simulink model "microgrid"  (R2023b)
settings: Solver=VariableStepAuto  StartTime=0.0  StopTime=10.0  RelTol=1e-3
libraries: simulink x10, spsThreePhaseSeriesRLCLoadLib x10, spsThreePhaseBreakerLib x10, spsThreePhaseVIMeasurementLib x6, spsGroundLib x6, eePowerMeasurement x4, spsControlledCurrentSourceLib x3, spsVariableInductorLib x3, spsVariableResistorLib x3, spsThreePhaseSeriesRLCBranchLib x2, spsAsynchronousMachinepuUnitsLib x1, spsThreePhaseTransformerTwoWindingsLib x1
settings Model: Creator=erandum  LastModifiedBy=erandum

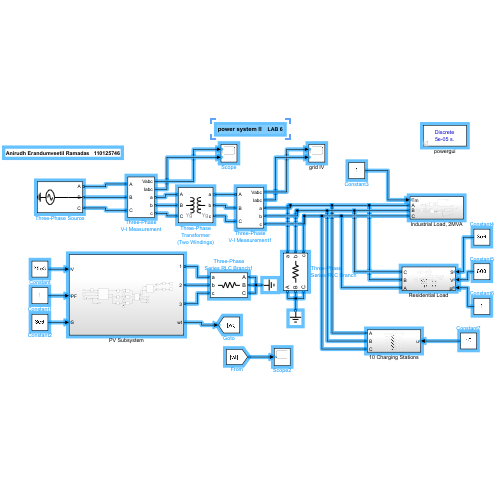
[thumbnail: Simulink's stored preview of the top-level diagram]
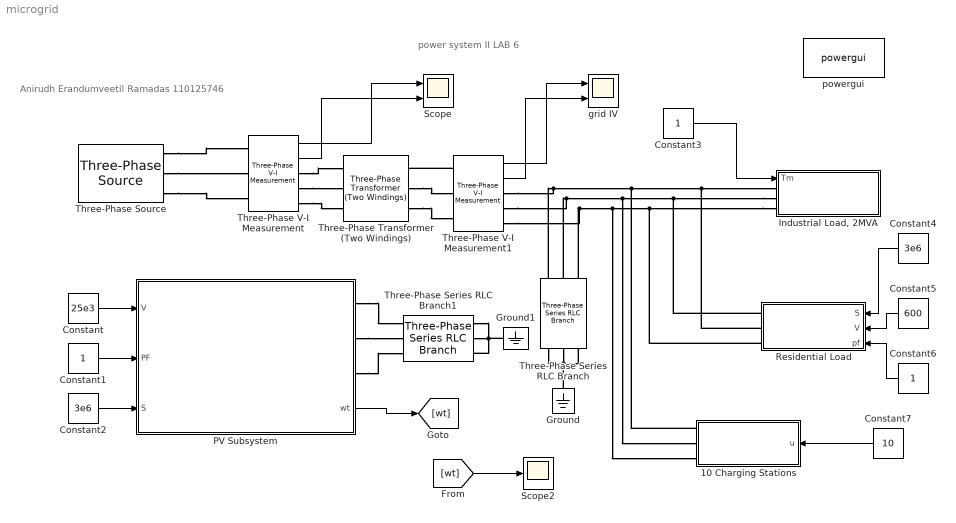
== system microgrid ==
  note: Anirudh Erandumveetil Ramadas 110125746
  note: power system II LAB 6
  10 Charging Stations : Subsystem
      settings: PortSchema="{\"entries\":[{\"content\":{\"sides\":[{\"content\":{\"connectorIds\":[\"LConn1\",\"LConn2\",\"LConn3\"]},\"type\":\"ConnectorPlacement.EquallySpacedRectSide\",\"uuid\":\"f1504b39-5c0e-4613-8c20-d8fb8d5da9a9\"},{\"content\":{\"connectorIds\":[\"In1\"],\"side\":\"RIGHT\"},\"type\":\"ConnectorPlacement.EquallySpacedRectSide\",\"uuid\":\"95b16e74-2cd8-4ce2-9ea5-c38ee840ee39\"},{\"content\":{\"side\":\"TOP\"},\"type\":\"ConnectorPlacement.EquallySpacedRectSide\",\"uuid\":\"c0d1c360-d2d5-4b2e-94da-07f0205a169d\"}]},\"type\":\"ConnectorPlacement.EquallySpacedConnector\",\"uuid\":\"27e98b22-6a64-4901-bf78-f4c065c24ca2\"}],\"packageUris\":[\"http://schema.mathworks.com/mf0/Connector/R2020b\"],\"version\":\"1.0\"}"
  Constant : Constant  Value=25e3
  Constant1 : Constant
  Constant2 : Constant  Value=3e6
  Constant3 : Constant
  Constant4 : Constant  Value=3e6
  Constant5 : Constant  Value=600
  Constant6 : Constant
  Constant7 : Constant  Value=10
  Ground : spsGroundLib/Ground  LConnTagsString=a
  Ground1 : spsGroundLib/Ground  LConnTagsString=a
  "Industrial Load, 2MVA" : Subsystem
  PV Subsystem : Subsystem
      settings: PortSchema="{\"entries\":[{\"content\":{\"sides\":[{\"content\":{\"connectorIds\":[\"In1\",\"In2\",\"In3\"]},\"type\":\"ConnectorPlacement.EquallySpacedRectSide\",\"uuid\":\"95cd3cc3-0877-4a04-ab5d-22b0c69ea079\"},{\"content\":{\"connectorIds\":[\"RConn1\",\"RConn2\",\"RConn3\",\"Out1\"],\"side\":\"RIGHT\"},\"type\":\"ConnectorPlacement.EquallySpacedRectSide\",\"uuid\":\"49167ea2-c585-4edc-b110-423b60a28fbc\"},{\"content\":{\"side\":\"TOP\"},\"type\":\"ConnectorPlacement.EquallySpacedRectSide\",\"uuid\":\"ee5ad331-2692-438a-a456-e1cd48d871f3\"}]},\"type\":\"ConnectorPlacement.EquallySpacedConnector\",\"uuid\":\"ab25702f-315c-43d0-b963-a7196bf7c14e\"}],\"packageUris\":[\"http://schema.mathworks.com/mf0/Connector/R2020b\"],\"version\":\"1.0\"}"
  Residential Load : Subsystem
      settings: PortSchema="{\"entries\":[{\"content\":{\"sides\":[{\"content\":{\"connectorIds\":[\"LConn1\",\"LConn2\",\"LConn3\"]},\"type\":\"ConnectorPlacement.EquallySpacedRectSide\",\"uuid\":\"1b5f4c68-a4bb-47ef-ac05-1fe32ae0a57a\"},{\"content\":{\"connectorIds\":[\"In1\",\"In2\",\"In3\"],\"side\":\"RIGHT\"},\"type\":\"ConnectorPlacement.EquallySpacedRectSide\",\"uuid\":\"b4b4f3e1-57b7-439b-8804-ae777d4c8250\"},{\"content\":{\"side\":\"TOP\"},\"type\":\"ConnectorPlacement.EquallySpacedRectSide\",\"uuid\":\"ef7d5d17-74d1-4089-bbe8-687aade085af\"}]},\"type\":\"ConnectorPlacement.EquallySpacedConnector\",\"uuid\":\"123b8064-54c2-4dec-b119-44036af93a53\"}],\"packageUris\":[\"http://schema.mathworks.com/mf0/Connector/R2020b\"],\"version\":\"1.0\"}"
  Scope : Scope  NumInputPorts=2
  Scope2 : Scope
  Three-Phase Series RLC Branch : spsThreePhaseSeriesRLCBranchLib/Three-Phase Series RLC Branch  LConnTagsString=A|B|C  RConnTagsString=A|B|C  BranchType=R  Resistance=1e6  Inductance=1e-3  Capacitance=1e-6  Measurements=None
  Three-Phase Series RLC Branch1 : spsThreePhaseSeriesRLCBranchLib/Three-Phase Series RLC Branch  LConnTagsString=A|B|C  RConnTagsString=A|B|C  BranchType=R  Resistance=1e6  Inductance=1e-3  Capacitance=1e-6  Measurements=None
  Three-Phase Transformer (Two Windings) : spsThreePhaseTransformerTwoWindingsLib/Three-Phase Transformer (Two Windings)  Winding1Connection=Yg  Winding2Connection=Yg  CoreType=Three single-phase transformers  SetSaturation=off  Hysteresis=off  DataFile='hysteresis'  SetInitialFlux=off  Measurements=None  UNITS=pu  NominalPower=[ 20e6 , 60 ]  Winding1=[ 25e3 , 0.002 , 0.08 ]  Winding2=[ 630 , 0.002 , 0.08 ]  Rm=500  Lm=500  L0=0.5  Saturation=[ 0,0 ; 0.0024,1.2 ; 1.0,1.52 ]  InitialFluxes=[ 0.8 , -0.8 , 0.7 ]  BreakLoop=off  DiscreteSolver=Trapezoidal iterative  DataType=off  TransfoNumber=1
  Three-Phase V-I Measurement : spsThreePhaseVIMeasurementLib/Three-Phase V-I Measurement  VoltageMeasurement=phase-to-ground  SetLabelV=off  LabelV=Vabc  Vpu=off  VpuLL=off  CurrentMeasurement=yes  SetLabelI=off  LabelI=Iabc  Ipu=off  Pbase=100e6  Vbase=500e3  OutputType=Complex  PhasorSimulation=off  PSBequivalent=0
  Three-Phase V-I Measurement1 : spsThreePhaseVIMeasurementLib/Three-Phase V-I Measurement  VoltageMeasurement=phase-to-ground  SetLabelV=off  LabelV=Vabc  Vpu=off  VpuLL=off  CurrentMeasurement=yes  SetLabelI=off  LabelI=Iabc  Ipu=off  Pbase=100e6  Vbase=500e3  OutputType=Complex  PhasorSimulation=off  PSBequivalent=0
  Three-Phase Source : spsThreePhaseSourceLib/Three-Phase Source  InternalConnection=Yg  VoltagePhases=off  Voltage=25e3  PhaseAngle=0  Voltage_phases=[25e3 25e3 25e3]/sqrt(3)  PhaseAngles_phases=[0 -120 +120]  Frequency=60  NonIdealSource=on  SpecifyImpedance=off  Resistance=0  Inductance=0  ShortCircuitLevel=100e6  BaseVoltage=25e3  XRratio=7  BusType=swing  Pref=10e3  Qref=0  Prefabc=[10e3, 10e3, 10e3]  Qrefabc=[0, 0, 0]  Qmin=-inf  Qmax=inf
  grid IV : Scope  NumInputPorts=2
  powergui : sps_lib/powergui  Priority=1  SimulationMode=Discrete  SampleTime=5e-05  frequency=60  Iterations=50  frequencyindice=0  Pbase=100e6  ErrMax=1e-4  UnitsV=kV  UnitsW=MW  buscounter=0  FunctionMessages=off  echomessages=off  EnableUseOfTLC=off  CurrentSourceSwitches=off  DisableSnubberDevices=off  DisableRonSwitches=off  DisableVfSwitches=off  DisplayEquations=off  AutomaticDiscreteSolvers=off  SolverType=Tustin/Backward Euler (TBE)  Interpol=off  ExternalGateDelay=off  methode=off  Ts=100  x0status=blocks  SPID=on  SwTol=0  HookPort=off  NonlinearTolerance=1e-4  nMaxIteration=100  ContinueOnMaxIteration=off  RestoreLinks=warning  ResistiveCurrentMeasurement=off  Frange=[0:2:500]  Ylog=off  Xlog=on  ShowGrid=off  save=off  variable=ZData  structure=0  ZoomFFT=off  StartTime=0.0  cycles=1  DisplayStyle=1  fundamental=60  FreqAxis=off  MaxFrequency=1000  frequencyindicesteady=1  RmsSteady=1  display=off
  wires:
  PV Subsystem/1(wt) -> [wt]
  Constant5/1 -> Residential Load/2(V)
  Constant3/1 -> "Industrial Load, 2MVA"/1(Tm)
  [wt] -> Scope2/1
  Constant4/1 -> Residential Load/1(S)
  Three-Phase V-I Measurement1/2 -> grid IV/2
  Three-Phase V-I Measurement1/1 -> grid IV/1
  Three-Phase V-I Measurement/2 -> Scope/2
  Constant7/1 -> 10 Charging Stations/1(u)
  Constant/1 -> PV Subsystem/1(V)
  Constant6/1 -> Residential Load/3(pf)
  Three-Phase V-I Measurement/1 -> Scope/1
  Constant2/1 -> PV Subsystem/3(S)
  Constant1/1 -> PV Subsystem/2(PF)
  connections:
  "Industrial Load, 2MVA"/LConn3 -- Three-Phase V-I Measurement1/RConn3 -- Three-Phase Series RLC Branch/RConn3 -- 10 Charging Stations/LConn3 -- Residential Load/LConn3
  "Industrial Load, 2MVA"/LConn2 -- Residential Load/LConn1 -- Three-Phase V-I Measurement1/RConn2 -- Three-Phase Series RLC Branch/RConn2 -- 10 Charging Stations/LConn2
  Three-Phase Series RLC Branch/RConn1 -- Three-Phase V-I Measurement1/RConn1 -- 10 Charging Stations/LConn1 -- Residential Load/LConn2 -- "Industrial Load, 2MVA"/LConn1
  Three-Phase Series RLC Branch/LConn2 -- Three-Phase Series RLC Branch/LConn1 -- Three-Phase Series RLC Branch/LConn3 -- Ground/LConn1
  Three-Phase Series RLC Branch1/LConn3 -- Three-Phase Series RLC Branch1/LConn1 -- Ground1/LConn1 -- Three-Phase Series RLC Branch1/LConn2
  PV Subsystem/RConn3 -- Three-Phase Series RLC Branch1/RConn3
  Three-Phase V-I Measurement/RConn1 -- Three-Phase Transformer (Two Windings)/LConn1
  PV Subsystem/RConn2 -- Three-Phase Series RLC Branch1/RConn2
  Three-Phase V-I Measurement/RConn2 -- Three-Phase Transformer (Two Windings)/LConn2
  Three-Phase Source/RConn3 -- Three-Phase V-I Measurement/LConn3
  Three-Phase V-I Measurement1/LConn1 -- Three-Phase Transformer (Two Windings)/RConn1
  Three-Phase Transformer (Two Windings)/RConn2 -- Three-Phase V-I Measurement1/LConn2
  Three-Phase Transformer (Two Windings)/RConn3 -- Three-Phase V-I Measurement1/LConn3
  Three-Phase Source/RConn1 -- Three-Phase V-I Measurement/LConn1
  PV Subsystem/RConn1 -- Three-Phase Series RLC Branch1/RConn1
  Three-Phase Source/RConn2 -- Three-Phase V-I Measurement/LConn2
  Three-Phase V-I Measurement/RConn3 -- Three-Phase Transformer (Two Windings)/LConn3

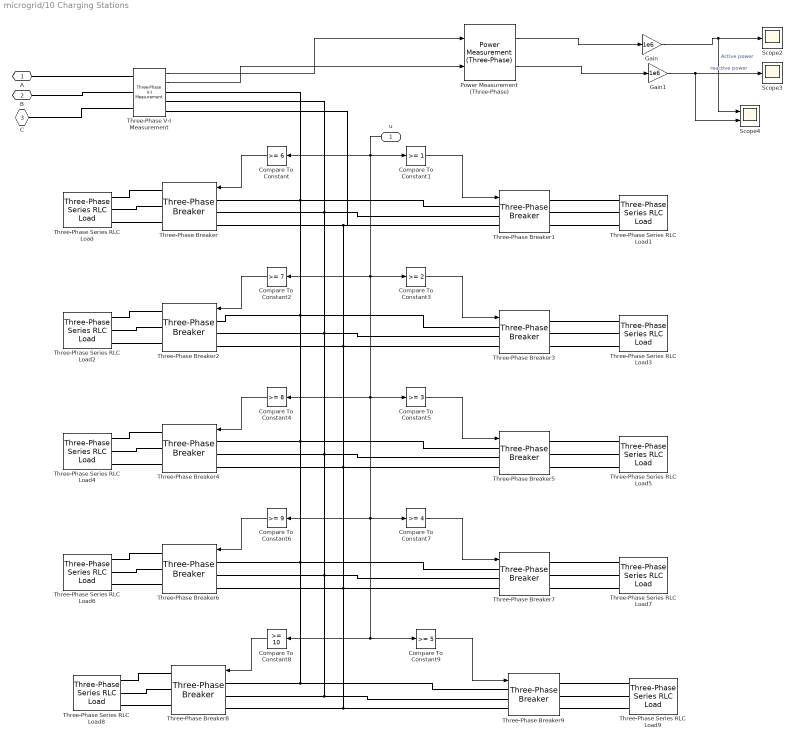
== system microgrid/10 Charging Stations ==
  u : Inport
  Compare To Constant : simulink/Logic and Bit Operations/Compare To Constant  relop=>=  const=6  OutDataTypeStr=boolean
  Compare To Constant1 : simulink/Logic and Bit Operations/Compare To Constant  relop=>=  const=1  OutDataTypeStr=boolean
  Compare To Constant2 : simulink/Logic and Bit Operations/Compare To Constant  relop=>=  const=7  OutDataTypeStr=boolean
  Compare To Constant3 : simulink/Logic and Bit Operations/Compare To Constant  relop=>=  const=2  OutDataTypeStr=boolean
  Compare To Constant4 : simulink/Logic and Bit Operations/Compare To Constant  relop=>=  const=8  OutDataTypeStr=boolean
  Compare To Constant5 : simulink/Logic and Bit Operations/Compare To Constant  relop=>=  const=3  OutDataTypeStr=boolean
  Compare To Constant6 : simulink/Logic and Bit Operations/Compare To Constant  relop=>=  const=9  OutDataTypeStr=boolean
  Compare To Constant7 : simulink/Logic and Bit Operations/Compare To Constant  relop=>=  const=4  OutDataTypeStr=boolean
  Compare To Constant8 : simulink/Logic and Bit Operations/Compare To Constant  relop=>=  const=10  OutDataTypeStr=boolean
  Compare To Constant9 : simulink/Logic and Bit Operations/Compare To Constant  relop=>=  const=5  OutDataTypeStr=boolean
  Gain : Gain  Gain=1e6
  Gain1 : Gain  Gain=1e6
  Power Measurement (Three-Phase) : eePowerMeasurement/Power Measurement (Three-Phase)  LabelModeActiveChoice=Continuous  F=60  K=[0 1 2 3]  Seq=Positive  Ts=0
  Scope2 : Scope
  Scope3 : Scope
  Scope4 : Scope  NumInputPorts=2
  Three-Phase Series RLC Load{,1..9} (10 alike) : spsThreePhaseSeriesRLCLoadLib/Three-Phase Series RLC Load  LConnTagsString=A|B|C  Configuration=Y (grounded)  NominalVoltage=600  Vabc=[1e3 1e3 1e3]  Vabcp=[1e3 1e3 1e3]  NominalFrequency=60  UnbalancedPower=off  ActivePower=400e3  InductivePower=0  CapacitivePower=0  Pabc=[10e3 9e3 11e3]  QLabc=[100 90 110]  QCabc=[100 90 110]  Pabcp=[10e3 9e3 11e3]  QLabcp=[100 90 110]  QCabcp=[100 90 110]  Measurements=None  LoadType=constant Z
  Three-Phase V-I Measurement : spsThreePhaseVIMeasurementLib/Three-Phase V-I Measurement  VoltageMeasurement=phase-to-ground  SetLabelV=off  LabelV=Vabc  Vpu=off  VpuLL=off  CurrentMeasurement=yes  SetLabelI=off  LabelI=Iabc  Ipu=off  Pbase=100e6  Vbase=500e3  OutputType=Complex  PhasorSimulation=off  PSBequivalent=0
  Three-Phase Breaker{,1..9} (10 alike) : spsThreePhaseBreakerLib/Three-Phase Breaker  InitialState=open  SwitchA=on  SwitchB=on  SwitchC=on  SwitchTimes="[1/60  5/60]"  External=on  BreakerResistance=0.01  SnubberResistance=1e6  SnubberCapacitance=inf  Measurements=None
  A : PMIOPort  Side=Left
  B : PMIOPort  Port=2  Side=Left
  C : PMIOPort  Port=3  Side=Left
  wires:
  Compare To Constant/1 -> Three-Phase Breaker/1
  Compare To Constant1/1 -> Three-Phase Breaker1/1
  Compare To Constant3/1 -> Three-Phase Breaker3/1
  Compare To Constant2/1 -> Three-Phase Breaker2/1
  Compare To Constant5/1 -> Three-Phase Breaker5/1
  Compare To Constant4/1 -> Three-Phase Breaker4/1
  Compare To Constant7/1 -> Three-Phase Breaker7/1
  Compare To Constant6/1 -> Three-Phase Breaker6/1
  Compare To Constant9/1 -> Three-Phase Breaker9/1
  Compare To Constant8/1 -> Three-Phase Breaker8/1
  u/1 -> Compare To Constant4/1, Compare To Constant5/1, Compare To Constant6/1, Compare To Constant7/1, Compare To Constant8/1, Compare To Constant9/1, Compare To Constant2/1, Compare To Constant3/1, Compare To Constant/1, Compare To Constant1/1
  Three-Phase V-I Measurement/1 -> Power Measurement (Three-Phase)/1
  Three-Phase V-I Measurement/2 -> Power Measurement (Three-Phase)/2
  Gain/1 -> Scope4/1, Scope2/1  "Active power"
  Gain1/1 -> Scope4/2, Scope3/1  "reactive power"
  Power Measurement (Three-Phase)/1 -> Gain/1
  Power Measurement (Three-Phase)/2 -> Gain1/1
  connections:
  A/RConn1 -- Three-Phase V-I Measurement/LConn1
  B/RConn1 -- Three-Phase V-I Measurement/LConn2
  C/RConn1 -- Three-Phase V-I Measurement/LConn3
  Three-Phase Series RLC Load/LConn1 -- Three-Phase Breaker/RConn1
  Three-Phase Series RLC Load/LConn2 -- Three-Phase Breaker/RConn2
  Three-Phase Series RLC Load/LConn3 -- Three-Phase Breaker/RConn3
  Three-Phase Breaker9/LConn1 -- Three-Phase Breaker8/LConn1 -- Three-Phase Breaker7/LConn1 -- Three-Phase Breaker2/LConn1 -- Three-Phase Breaker3/LConn1 -- Three-Phase V-I Measurement/RConn1 -- Three-Phase Breaker/LConn1 -- Three-Phase Breaker1/LConn1 -- Three-Phase Breaker4/LConn1 -- Three-Phase Breaker5/LConn1 -- Three-Phase Breaker6/LConn1
  Three-Phase Breaker9/LConn2 -- Three-Phase Breaker8/LConn2 -- Three-Phase Breaker6/LConn2 -- Three-Phase Breaker7/LConn2 -- Three-Phase Breaker4/LConn2 -- Three-Phase Breaker5/LConn2 -- Three-Phase Breaker2/LConn2 -- Three-Phase Breaker3/LConn2 -- Three-Phase V-I Measurement/RConn2 -- Three-Phase Breaker/LConn2 -- Three-Phase Breaker1/LConn2
  Three-Phase Breaker9/LConn3 -- Three-Phase Breaker8/LConn3 -- Three-Phase Breaker6/LConn3 -- Three-Phase Breaker7/LConn3 -- Three-Phase Breaker4/LConn3 -- Three-Phase Breaker5/LConn3 -- Three-Phase Breaker/LConn3 -- Three-Phase V-I Measurement/RConn3 -- Three-Phase Breaker1/LConn3 -- Three-Phase Breaker2/LConn3 -- Three-Phase Breaker3/LConn3
  Three-Phase Series RLC Load1/LConn1 -- Three-Phase Breaker1/RConn1
  Three-Phase Series RLC Load1/LConn2 -- Three-Phase Breaker1/RConn2
  Three-Phase Series RLC Load1/LConn3 -- Three-Phase Breaker1/RConn3
  Three-Phase Series RLC Load3/LConn2 -- Three-Phase Breaker3/RConn2
  Three-Phase Series RLC Load2/LConn2 -- Three-Phase Breaker2/RConn2
  Three-Phase Series RLC Load3/LConn3 -- Three-Phase Breaker3/RConn3
  Three-Phase Series RLC Load3/LConn1 -- Three-Phase Breaker3/RConn1
  Three-Phase Series RLC Load2/LConn1 -- Three-Phase Breaker2/RConn1
  Three-Phase Series RLC Load2/LConn3 -- Three-Phase Breaker2/RConn3
  Three-Phase Series RLC Load5/LConn2 -- Three-Phase Breaker5/RConn2
  Three-Phase Series RLC Load4/LConn2 -- Three-Phase Breaker4/RConn2
  Three-Phase Series RLC Load5/LConn3 -- Three-Phase Breaker5/RConn3
  Three-Phase Series RLC Load5/LConn1 -- Three-Phase Breaker5/RConn1
  Three-Phase Series RLC Load4/LConn1 -- Three-Phase Breaker4/RConn1
  Three-Phase Series RLC Load4/LConn3 -- Three-Phase Breaker4/RConn3
  Three-Phase Series RLC Load7/LConn2 -- Three-Phase Breaker7/RConn2
  Three-Phase Series RLC Load6/LConn2 -- Three-Phase Breaker6/RConn2
  Three-Phase Series RLC Load7/LConn3 -- Three-Phase Breaker7/RConn3
  Three-Phase Series RLC Load7/LConn1 -- Three-Phase Breaker7/RConn1
  Three-Phase Series RLC Load6/LConn1 -- Three-Phase Breaker6/RConn1
  Three-Phase Series RLC Load6/LConn3 -- Three-Phase Breaker6/RConn3
  Three-Phase Series RLC Load9/LConn2 -- Three-Phase Breaker9/RConn2
  Three-Phase Series RLC Load8/LConn2 -- Three-Phase Breaker8/RConn2
  Three-Phase Series RLC Load9/LConn3 -- Three-Phase Breaker9/RConn3
  Three-Phase Series RLC Load9/LConn1 -- Three-Phase Breaker9/RConn1
  Three-Phase Series RLC Load8/LConn1 -- Three-Phase Breaker8/RConn1
  Three-Phase Series RLC Load8/LConn3 -- Three-Phase Breaker8/RConn3

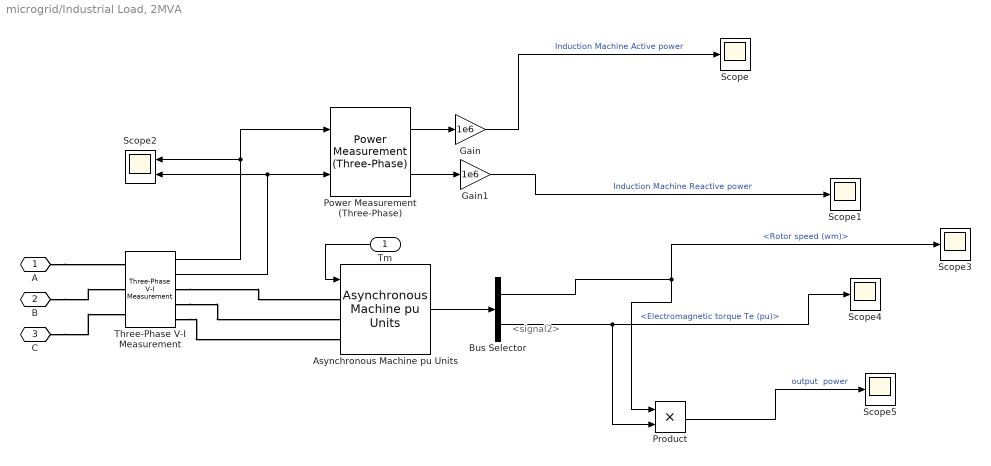
== system microgrid/Industrial Load, 2MVA ==
  note: <signal2>
  Tm : Inport
  Asynchronous Machine pu Units : spsAsynchronousMachinepuUnitsLib/Asynchronous Machine pu Units  RotorType=Squirrel-cage  PresetModel=No  MechanicalLoad=Torque Tm  ShowDetailedParameters=on  ReferenceFrame=Rotor  Units=pu  MeasurementBus=off  NominalParameters=[2e6 600 60]  VoltageRatio=1  Stator=[0.006 0.04832]  Rotor=[0.01909 0.0397]  Cage1=[0.01909 0.0397]  Cage2=[0.01909 0.0397]  Lm=1  Mechanical=[0.3096 0.01511 2]  PolePairs=2  InitialConditions="[ 1,0   0,0,0   0,0,0 ]"  SimulateSaturation=off  Saturation="[0.212,0.4201,0.8125,1.0979,1.4799,2.2457,3.2586,4.5763,6.4763 ;   0.5,0.7,0.9,1,1.1,1.2 ,1.3,1.4,1.5]"  LoadFlowParameters=0  TsPowergui=0  TsBlock=-1  IterativeModel=Trapezoidal non iterative  IterativeDiscreteModel=Trapezoidal non iterative  Pmec=0
      settings: LibrarySourceBlock=|
      | sps_lib/Electrical Machines/Asynchronous Machine
      | pu Units
  Bus Selector : BusSelector  OutputSignals=Mechanical.Rotor speed (wm),Mechanical.Electromagnetic torque Te (pu)
  Gain : Gain  Gain=1e6
  Gain1 : Gain  Gain=1e6
  Power Measurement (Three-Phase) : eePowerMeasurement/Power Measurement (Three-Phase)  LabelModeActiveChoice=Continuous  F=60  K=[0 1 2 3]  Seq=Positive  Ts=0
  Product : Product
  Scope{,1,3..5} (5 alike) : Scope
  Scope2 : Scope  NumInputPorts=2
  Three-Phase V-I Measurement : spsThreePhaseVIMeasurementLib/Three-Phase V-I Measurement  VoltageMeasurement=phase-to-ground  SetLabelV=off  LabelV=Vabc  Vpu=off  VpuLL=off  CurrentMeasurement=yes  SetLabelI=off  LabelI=Iabc  Ipu=off  Pbase=100e6  Vbase=500e3  OutputType=Complex  PhasorSimulation=off  PSBequivalent=0
  A : PMIOPort  Side=Left
  B : PMIOPort  Port=2  Side=Left
  C : PMIOPort  Port=3  Side=Left
  wires:
  Three-Phase V-I Measurement/1 -> Scope2/1, Power Measurement (Three-Phase)/1
  Three-Phase V-I Measurement/2 -> Scope2/2, Power Measurement (Three-Phase)/2
  Power Measurement (Three-Phase)/1 -> Gain/1
  Power Measurement (Three-Phase)/2 -> Gain1/1
  Gain/1 -> Scope/1  "Induction Machine Active power"
  Gain1/1 -> Scope1/1  "Induction Machine Reactive power"
  Tm/1 -> Asynchronous Machine pu Units/1
  Asynchronous Machine pu Units/1 -> Bus Selector/1
  Bus Selector/1 -> Product/1, Scope3/1  "<Rotor speed (wm)>"
  Product/1 -> Scope5/1  "output  power"
  Bus Selector/2 -> Product/2, Scope4/1  "<Electromagnetic torque Te (pu)>"
  connections:
  A/RConn1 -- Three-Phase V-I Measurement/LConn1
  B/RConn1 -- Three-Phase V-I Measurement/LConn2
  C/RConn1 -- Three-Phase V-I Measurement/LConn3
  Three-Phase V-I Measurement/RConn1 -- Asynchronous Machine pu Units/LConn1
  Three-Phase V-I Measurement/RConn2 -- Asynchronous Machine pu Units/LConn2
  Three-Phase V-I Measurement/RConn3 -- Asynchronous Machine pu Units/LConn3

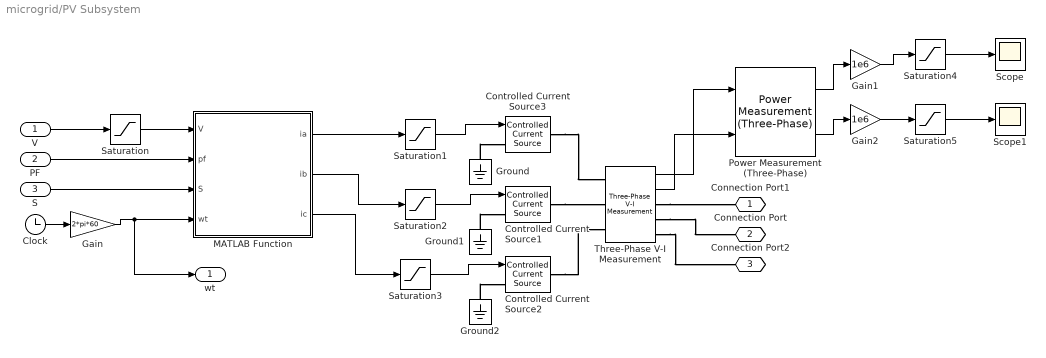
== system microgrid/PV Subsystem ==
  V : Inport
  PF : Inport  Port=2
  S : Inport  Port=3
  Clock : Clock
  Controlled Current Source1 : spsControlledCurrentSourceLib/Controlled Current Source  Initialize=on  Source_Type=AC  Amplitude=0  Phase=0  Frequency=0  Measurements=None
  Controlled Current Source2 : spsControlledCurrentSourceLib/Controlled Current Source  Initialize=on  Source_Type=AC  Amplitude=0  Phase=0  Frequency=0  Measurements=None
  Controlled Current Source3 : spsControlledCurrentSourceLib/Controlled Current Source  Initialize=on  Source_Type=AC  Amplitude=0  Phase=0  Frequency=0  Measurements=None
  Gain : Gain  Gain=2*pi*60
  Gain1 : Gain  Gain=1e6
  Gain2 : Gain  Gain=1e6
  Ground : spsGroundLib/Ground  LConnTagsString=a
  Ground1 : spsGroundLib/Ground  LConnTagsString=a
  Ground2 : spsGroundLib/Ground  LConnTagsString=a
  MATLAB Function : MATLAB Function  TreatAsAtomicUnit=on
  Power Measurement (Three-Phase) : eePowerMeasurement/Power Measurement (Three-Phase)  LabelModeActiveChoice=Continuous  F=60  K=[0 1 2 3]  Seq=Positive  Ts=0
  Saturation : Saturate
  Saturation1 : Saturate  UpperLimit=700  LowerLimit=-700
  Saturation2 : Saturate
  Saturation3 : Saturate
  Saturation4 : Saturate  UpperLimit=5e6  LowerLimit=-5e6
  Saturation5 : Saturate  UpperLimit=5e6  LowerLimit=-5e6
  Scope : Scope
  Scope1 : Scope
  Three-Phase V-I Measurement : spsThreePhaseVIMeasurementLib/Three-Phase V-I Measurement  VoltageMeasurement=phase-to-ground  SetLabelV=off  LabelV=Vabc  Vpu=off  VpuLL=off  CurrentMeasurement=yes  SetLabelI=off  LabelI=Iabc  Ipu=off  Pbase=100e6  Vbase=500e3  OutputType=Complex  PhasorSimulation=off  PSBequivalent=0
  Connection Port1 : PMIOPort  Side=Right
  Connection Port : PMIOPort  Port=2  Side=Right
  Connection Port2 : PMIOPort  Port=3  Side=Right
  wt : Outport
  wires:
  Saturation5/1 -> Scope1/1
  Power Measurement (Three-Phase)/2 -> Gain2/1
  Saturation/1 -> MATLAB Function/1(V)
  Saturation4/1 -> Scope/1
  Saturation3/1 -> Controlled Current Source2/1
  Power Measurement (Three-Phase)/1 -> Gain1/1
  Gain/1 -> wt/1, MATLAB Function/4(wt)
  Gain1/1 -> Saturation4/1
  Three-Phase V-I Measurement/2 -> Power Measurement (Three-Phase)/2
  Saturation2/1 -> Controlled Current Source1/1
  MATLAB Function/3(ic) -> Saturation3/1
  Three-Phase V-I Measurement/1 -> Power Measurement (Three-Phase)/1
  V/1 -> Saturation/1
  Clock/1 -> Gain/1
  MATLAB Function/1(ia) -> Saturation1/1
  S/1 -> MATLAB Function/3(S)
  Saturation1/1 -> Controlled Current Source3/1
  PF/1 -> MATLAB Function/2(pf)
  Gain2/1 -> Saturation5/1
  MATLAB Function/2(ib) -> Saturation2/1
  connections:
  Ground/LConn1 -- Controlled Current Source3/LConn1
  Ground1/LConn1 -- Controlled Current Source1/LConn1
  Controlled Current Source2/RConn1 -- Three-Phase V-I Measurement/LConn3
  Ground2/LConn1 -- Controlled Current Source2/LConn1
  Controlled Current Source3/RConn1 -- Three-Phase V-I Measurement/LConn1
  Controlled Current Source1/RConn1 -- Three-Phase V-I Measurement/LConn2
  Three-Phase V-I Measurement/RConn1 -- Connection Port1/RConn1
  Three-Phase V-I Measurement/RConn2 -- Connection Port/RConn1
  Three-Phase V-I Measurement/RConn3 -- Connection Port2/RConn1

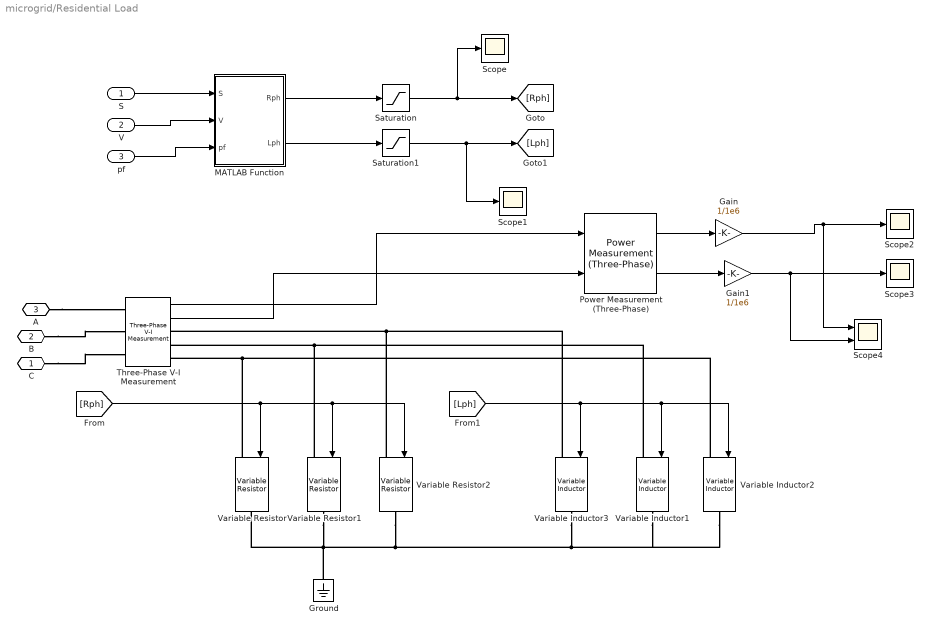
== system microgrid/Residential Load ==
  S : Inport
  V : Inport  Port=2
  pf : Inport  Port=3
  Gain : Gain  Gain=1/1e6
  Gain1 : Gain  Gain=1/1e6
  Ground : spsGroundLib/Ground  LConnTagsString=a
  MATLAB Function : MATLAB Function  TreatAsAtomicUnit=on
  Power Measurement (Three-Phase) : eePowerMeasurement/Power Measurement (Three-Phase)  LabelModeActiveChoice=Continuous  F=60  K=[0 1 2 3]  Seq=Positive  Ts=0
  Saturation : Saturate  UpperLimit=1e6  LowerLimit=0
  Saturation1 : Saturate  UpperLimit=1e6  LowerLimit=0
  Scope{,1..3} (4 alike) : Scope
  Scope4 : Scope  NumInputPorts=2
  Three-Phase V-I Measurement : spsThreePhaseVIMeasurementLib/Three-Phase V-I Measurement  VoltageMeasurement=phase-to-ground  SetLabelV=off  LabelV=Vabc  Vpu=off  VpuLL=off  CurrentMeasurement=yes  SetLabelI=off  LabelI=Iabc  Ipu=off  Pbase=100e6  Vbase=500e3  OutputType=Complex  PhasorSimulation=off  PSBequivalent=0
  Variable Inductor1 : spsVariableInductorLib/Variable Inductor  methode=Backward Euler  Labsmin=1e-6  Initialize=off  iL0=0  L0=1e-3  Vl0=-0.080237
      settings: LibrarySourceBlock=sps_lib/Passives/Variable Inductor
  Variable Inductor2 : spsVariableInductorLib/Variable Inductor  methode=Backward Euler  Labsmin=1e-6  Initialize=off  iL0=0  L0=1e-3  Vl0=-445.3641
      settings: LibrarySourceBlock=sps_lib/Passives/Variable Inductor
  Variable Inductor3 : spsVariableInductorLib/Variable Inductor  methode=Backward Euler  Labsmin=1e-6  Initialize=off  iL0=0  L0=1e-3  Vl0=445.4443
      settings: LibrarySourceBlock=sps_lib/Passives/Variable Inductor
  Variable Resistor : spsVariableResistorLib/Variable Resistor  Rabsmin=1e-3
      settings: LibrarySourceBlock=sps_lib/Passives/Variable Resistor
  Variable Resistor1 : spsVariableResistorLib/Variable Resistor  Rabsmin=1e-3
      settings: LibrarySourceBlock=sps_lib/Passives/Variable Resistor
  Variable Resistor2 : spsVariableResistorLib/Variable Resistor  Rabsmin=1e-3
      settings: LibrarySourceBlock=sps_lib/Passives/Variable Resistor
  C : PMIOPort  Side=Left
  B : PMIOPort  Port=2  Side=Left
  A : PMIOPort  Port=3  Side=Left
  wires:
  S/1 -> MATLAB Function/1(S)
  V/1 -> MATLAB Function/2(V)
  pf/1 -> MATLAB Function/3(pf)
  MATLAB Function/1(Rph) -> Saturation/1
  MATLAB Function/2(Lph) -> Saturation1/1
  Saturation/1 -> Scope/1, [Rph]
  Saturation1/1 -> Scope1/1, [Lph]
  [Rph] -> Variable Resistor1/1, Variable Resistor2/1, Variable Resistor/1
  [Lph] -> Variable Inductor2/1, Variable Inductor1/1, Variable Inductor3/1
  Three-Phase V-I Measurement/1 -> Power Measurement (Three-Phase)/1
  Three-Phase V-I Measurement/2 -> Power Measurement (Three-Phase)/2
  Power Measurement (Three-Phase)/1 -> Gain/1
  Power Measurement (Three-Phase)/2 -> Gain1/1
  Gain/1 -> Scope4/1, Scope2/1
  Gain1/1 -> Scope4/2, Scope3/1
  connections:
  A/RConn1 -- Three-Phase V-I Measurement/LConn1
  B/RConn1 -- Three-Phase V-I Measurement/LConn2
  C/RConn1 -- Three-Phase V-I Measurement/LConn3
  Variable Inductor2/LConn1 -- Variable Resistor/LConn1 -- Three-Phase V-I Measurement/RConn3
  Variable Inductor1/LConn1 -- Variable Resistor1/LConn1 -- Three-Phase V-I Measurement/RConn2
  Variable Inductor3/LConn1 -- Variable Resistor2/LConn1 -- Three-Phase V-I Measurement/RConn1
  Variable Resistor1/RConn1 -- Variable Inductor2/RConn1 -- Variable Inductor1/RConn1 -- Variable Inductor3/RConn1 -- Variable Resistor2/RConn1 -- Ground/LConn1 -- Variable Resistor/RConn1

== matlab function microgrid/Residential Load/MATLAB Function ==
  data: S input; Rph output; V input; pf input; Lph output
function [Rph, Lph] = fcn(S, V, pf)

Theta= acos(pf);
P3p= S*cos(Theta);
Q3p= S*sin(Theta);

Rph = 3*(V)^2/P3p;
Xph = 3*(V)^2/Q3p;
Lph = Xph/(2*pi*60);

return

== matlab function microgrid/PV Subsystem/MATLAB Function ==
  data: V input; pf input; S input; ia output; wt input; ib output; ic output
function [ia, ib, ic]=fcn(V, pf, S, wt)

Theta=1*acos (pf);

I=sqrt(2/3)*(S/V);

ia=I*sin(wt-Theta);

ib=I*sin(wt-Theta-2*pi/3);

ic=I*sin(wt-Theta+2*pi/3);

return;
